simulink model "Pong3D"  (R2016b)
settings: Solver=ode45  StartTime=0.0  StopTime=10.0  FixedStep=0.001  MaxStep=updateFrequency  RelTol=1e-3  EnableMultiTasking=on
values from neighbouring files (symbols this model uses):
  Ball = struct(B_field1,B_value1,B_field2,B_value2,B_field3,B_value3,     B_field4,B_value4,B_field5,B_value5)    [PingPongStructs6DOF.m]
  Contact_Forces = struct(CF_field1,CF_value1,CF_field2,CF_value2,CF_field3,CF_value3)    [PingPongStructs6DOF.m]
  g = 9.81    [PingPongStructs6DOF.m]
  m = V(2)/V(1)    [AIPlayer.m]
  Net = struct(N_field1,N_value1)    [PingPongStructs6DOF.m]
  Robot1 = struct(R1_field1,R1_value1,R1_field2,R1_value2,R1_field3,R1_value3,     R1_field4,R1_value4, R1_field5,R1_value5,R1_field6,R1_value6,     R1_field7,R1_value7,R1_field8,R1_value8,R1_field9,R1_value9,R1_field10,R1_value10,     R1_field11,R1_value11,R1_field12,R1_value12)    [PingPongStructs6DOF.m]
  Robot2 = struct(R2_field1,R2_value1,R2_field2,R2_value2,R2_field3,R2_value3,     R2_field4, R2_value4, R2_field5,R2_value5,R2_field6,R2_value6,     R2_field7, R2_value7, R2_field8, R2_value8, R2_field9, R2_value9, R2_field10, R2_value10,     R2_field11, R2_value11, R2_field12, R2_value12)    [PingPongStructs6DOF.m]
  Table = struct(T_field1,T_value1,T_field2,T_value2)    [PingPongStructs6DOF.m]
undefined symbols (not defined in the file or in its folder): X, Y, Z
libraries: sm_lib x120, nesl_utility x55, fl_lib x48, Contact_Forces_Lib x4, Parts_Lib x3
(part 5 of 5)

== system Pong3D/Robot 2/Joint6/Limit Joint 4 Y ==
  Ideal Angular Velocity Source : fl_lib/Mechanical/Mechanical Sources/Ideal Angular Velocity Source
  Ideal Torque Sensor : fl_lib/Mechanical/Mechanical Sensors/Ideal Torque Sensor
  Mechanical Rotational Reference : fl_lib/Mechanical/Rotational Elements/Mechanical Rotational Reference
  Rotational Hard Stop1 : fl_lib/Mechanical/Rotational Elements/Rotational Hard Stop  upper_bnd=Robot2.Joint.Upper_Bound(6) - Robot2.Joint.Initial_Angle(6) deg  lower_bnd=Robot2.Joint.Lower_Bound(6) - Robot2.Joint.Initial_Angle(6) deg  stiff_up=Robot2.Joint.Contact_Stiffness(6) N*m/rad  stiff_low=Robot2.Joint.Contact_Stiffness(6) N*m/rad  D_up=Robot2.Joint.Contact_Damping(6) N*m/(rad/s)  D_low=Robot2.Joint.Contact_Damping(6) N*m/(rad/s)  w_specify=off  w_priority=High  w=0 rad/s  t_specify=off  t_priority=High  t=0 N*m  phi_specify=off  phi_priority=High  phi=0 rad
  T : PMIOPort  Port=1  Side=Right
  W : PMIOPort  Port=2  Side=Left
  connections:
  Ideal Torque Sensor/LConn1 -- Ideal Angular Velocity Source/RConn2
  Ideal Torque Sensor/RConn2 -- T/RConn1
  Rotational Hard Stop1/RConn1 -- Ideal Torque Sensor/RConn1
  Rotational Hard Stop1/LConn1 -- Mechanical Rotational Reference/LConn1 -- Ideal Angular Velocity Source/LConn1
  W/RConn1 -- Ideal Angular Velocity Source/RConn1
